simulink library "peripheral_utilities"  (R2024b)
settings: Solver=VariableStepAuto  StartTime=0.0  StopTime=10.0  RelTol=1e-3
libraries: $bdroot x19, simulink x5, spsSeriesRLCBranchLib x3, spsVoltageMeasurementLib x2, spsMosfetLib x2, spsCurrentMeasurementLib x1, spsSecondOrderFilterLib x1, spsGroundLib x1
(part 1 of 2)
settings Model: Creator=Javnson  LastModifiedBy=javnson
settings OptimizationCC: ReuseModelBlockBuffer=off
settings RTWCC: GPUComputeCapability=3.5

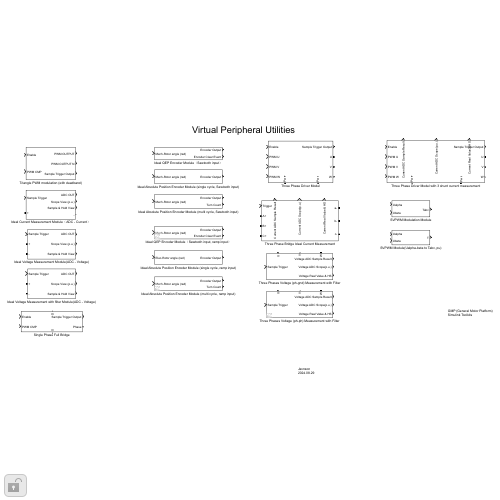
[thumbnail: Simulink's stored preview of the top-level diagram]
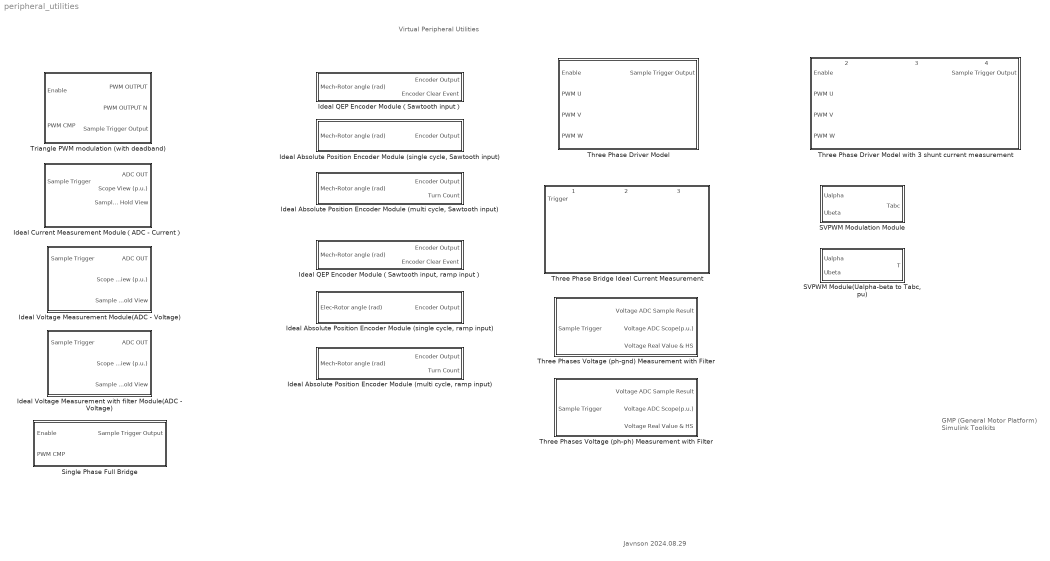
== system peripheral_utilities ==
  note: Virtual Peripheral Utilities
  note: GMP (General Motor Platform)
      | Simulink Toolkits
  note: Javnson
      | 2024.08.29
  "Ideal Absolute Position Encoder Module (multi cycle, Sawtooth input)" : Subsystem  mask{ENCODER_BIT=17}
      mask DialogControl DescGroupVar Prompt: Ideal Absolute Position Encoder Module (multi cycle, Sawtooth input)
      mask DialogControl DescTextVar Prompt: Avsolute Encoder transfer a motor mechanical angle (thetam, rad) to Absolute Encoder result. Generally, an absolute encoder has 17-bits or 23-bits resolution results.
      mask DialogControl Control3 Prompt: GMP CTL Simulink Utilities: virtual peripherals
      mask DialogControl ParameterGroupVar Prompt: 参数
      mask DialogControl Control2 Prompt: Absolute Encoder Resolution (bits):
  "Ideal Absolute Position Encoder Module (multi cycle, ramp input)" : Subsystem  AncestorBlock=peripheral_utilities/Ideal Absolute Position Encoder Module (multi cycle, Sawtooth input)  mask{ENCODER_BIT=17}
      mask DialogControl DescGroupVar Prompt: Ideal Absolute Position Encoder Module (multi cycle, Sawtooth input)
      mask DialogControl Control3 Prompt: GMP CTL Simulink Utilities: virtual peripherals
      mask DialogControl DescTextVar Prompt: Avsolute Encoder transfer a motor mechanical angle (thetam, rad) to Absolute Encoder result. Generally, an absolute encoder has 17-bits or 23-bits resolution results.
      mask DialogControl ParameterGroupVar Prompt: 参数
      mask DialogControl Control2 Prompt: Absolute Encoder Resolution (bits):
  "Ideal Absolute Position Encoder Module (single cycle, Sawtooth input)" : Subsystem  mask{ENCODER_BIT=17}
      mask DialogControl DescGroupVar Prompt: Ideal Absolute Position Encoder Module (single cycle, Sawtooth input)
      mask DialogControl DescTextVar Prompt: Avsolute Encoder transfer a motor angle (thetam, rad) to Absolute Encoder result. Generally, an absolute encoder has 17-bits or 23-bits resolution results.
      mask DialogControl Control3 Prompt: GMP CTL Simulink Utilities: virtual peripherals
      mask DialogControl ParameterGroupVar Prompt: parameters
      mask DialogControl Control2 Prompt: Absolute Encoder Resolution (bits):
  "Ideal Absolute Position Encoder Module (single cycle, ramp input)" : Subsystem  mask{ENCODER_BIT=17}
      mask DialogControl DescGroupVar Prompt: Ideal Absolute Position Encoder Module (single cycle)
      mask DialogControl DescTextVar Prompt: Avsolute Encoder transfer a motor mechanical angle (thetam, rad) to Absolute Encoder result. Generally, an absolute encoder has 17-bits or 23-bits resolution results.
      mask DialogControl Control3 Prompt: GMP CTL Simulink Utilities: virtual peripherals
      mask DialogControl ParameterGroupVar Prompt: 参数
      mask DialogControl Control2 Prompt: Absolute Encoder Resolution (bits):
  Ideal Current Measurement Module（ADC - Current） : Subsystem  mask{ADC_GAIN=1, ADC_BIT=16, ADC_REFERENCE=20.0, ADC_BIAS=10, ADC_INIT=0}
      mask DialogControl DescGroupVar Prompt: Current Sample ADC Model 1
      mask DialogControl DescTextVar Prompt: This is a ideal Current Measurement Module. This module enable a bias and a gain, and finally output a ADC result.
      mask DialogControl Control8 Prompt: ADC(p.u.) = (real_current * ADC_GAIN + ADC_BIAS)/ADC_REFERENCE
      mask DialogControl Control9 Prompt: GMP CTL Simulink Utilities: virtual peripherals
      mask DialogControl ParameterGroupVar Prompt: 参数
      mask DialogControl Control7 Prompt: ADC Current Gain (Scale Factor):
      mask DialogControl Control2 Prompt: ADC resolution:
      mask DialogControl Control4 Prompt: ADC reference Current(A), ADC full scale current (when gain = 1)
      mask DialogControl Control5 Prompt: ADC Bias Current(A)
      mask DialogControl Control6 Prompt: ADC initial Current Output(A)
  "Ideal QEP Encoder Module（Sawtooth input, ramp input）" : Subsystem  AncestorBlock=peripheral_utilities/Ideal QEP Encoder Module（Sawtooth input）  mask{QEP_LINE=2000}
      mask DialogControl DescGroupVar Prompt: Ideal QEP Encoder Module
      mask DialogControl DescTextVar Prompt: QEP encoder transfer a motor mechanical angle (thetam, rad) to QEP encoder results. The maximum output is 4 * QEP_LINE and generate a reseet event each round.
      mask DialogControl Control4 Prompt: GMP CTL Simulink Utilities: virtual peripherals
      mask DialogControl ParameterGroupVar Prompt: 参数
      mask DialogControl Control3 Prompt: QEP encoder lines count:
  Ideal QEP Encoder Module（Sawtooth input） : Subsystem  mask{QEP_LINE=2000}
      mask DialogControl DescGroupVar Prompt: Ideal QEP Encoder Module
      mask DialogControl DescTextVar Prompt: QEP encoder transfer a motor mechanical angle (thetam, rad) to QEP encoder results. The maximum output is 4 * QEP_LINE and generate a reseet event each round.
      mask DialogControl Control4 Prompt: GMP CTL Simulink Utilities: virtual peripherals
      mask DialogControl ParameterGroupVar Prompt: 参数
      mask DialogControl Control3 Prompt: QEP encoder lines count:
  Ideal Voltage Measurement Module(ADC - Voltage) : Subsystem  mask{ADC_GAIN=1/10, ADC_BIT=16, ADC_REFERENCE=3, ADC_BIAS=0, ADC_INIT=0}
      mask DialogControl DescGroupVar Prompt: Voltage Sample ADC Model
      mask DialogControl DescTextVar Prompt: This is a ideal Voltage Measurement Module.
      mask DialogControl Control2 Prompt: ADC(p.u.) = (real_voltage * ADC_GAIN + ADC_BIAS)/ADC_REFERENCE
      mask DialogControl Control9 Prompt: GMP CTL Simulink Utilities: virtual peripherals
      mask DialogControl ParameterGroupVar Prompt: Parameters:
      mask DialogControl Control4 Prompt: ADC Voltage Gain (Scale Factor):
      mask DialogControl Control5 Prompt: ADC resolution:
      mask DialogControl Control6 Prompt: ADC reference Voltage(V)
      mask DialogControl Control8 Prompt: ADC Bias Voltage(V)
      mask DialogControl Control7 Prompt: ADC Initial Voltage Output (V):
  Ideal Voltage Measurement with filter Module(ADC - Voltage) : Subsystem  mask{ADC_GAIN=1, ADC_BIT=16, ADC_REFERENCE=3, ADC_BIAS=0, ADC_INIT=0, cut_frequency=500}
      mask DialogControl DescGroupVar Prompt: Voltage Sample ADC Model
      mask DialogControl DescTextVar Prompt: This is a ideal Voltage Measurement Module.
      mask DialogControl Control2 Prompt: ADC(p.u.) = (real_voltage * ADC_GAIN + ADC_BIAS)/ADC_REFERENCE
      mask DialogControl Control11 Prompt: GMP CTL Simulink Utilities: virtual peripherals
      mask DialogControl ParameterGroupVar Prompt: Parameters:
      mask DialogControl Control4 Prompt: ADC Voltage Gain (Scale Factor):
      mask DialogControl Control5 Prompt: ADC resolution:
      mask DialogControl Control6 Prompt: ADC reference Voltage(V)
      mask DialogControl Control8 Prompt: ADC Bias Voltage(V)
      mask DialogControl Control7 Prompt: ADC Initial Voltage Output (V):
      mask DialogControl Control9 Prompt: Voltage Filter cut frequency (Hz):
      mask DialogControl Control10 Prompt: Generally, this value less than switch frequency / 10, greater than motor normal frequency * 3
  SVPWM Modulation Module : Subsystem  mask{half_cmp=10000}
      mask DialogControl DescGroupVar Prompt: SVPWM Modulation
      mask DialogControl DescTextVar Prompt: This Module Provide a dual level svpwm modulation tools.
      mask DialogControl Control4 Prompt: GMP CTL Simulink Utilities: virtual peripherals
      mask DialogControl Control3 Prompt: EPWM module Half Compare
  "SVPWM Module(Ualpha-beta to Tabc, pu)" : Subsystem  mask{half_cycle=10000}
      mask prompts: half_cycle "Half cycle"
      mask DialogControl DescGroupVar Prompt: SVPWM to Tabc
      mask DialogControl DescTextVar Prompt: GMP CTL Simulink Utilities: virtual peripherals
      mask DialogControl Control2 Prompt: SVPWM modulation module. Output is the compare register value.
      mask DialogControl ParameterGroupVar Prompt: Parameters:
      mask DialogControl Control3 Prompt: SVPWM Modulation Half cycle:
  Single Phase Full Bridge : Subsystem  mask{fswitch=10e3, CMP_MAX=10000, Deadband_Upper=100, Deadband_Lower=100, Deadband_us=1, phase_shift=0, R_mosfet_on=0.1, Lon=0, Rd=0.01, Vf=0.3, Rs=1e5, Cs=inf}
      mask init:
      | calculate_deadband(gcb, 'Deadband_Upper', 'Deadband_Lower',	'CMP_MAX', 'fswitch', 'Deadband_us');
      settings: PortSchema="{\"entries\":[{\"content\":{\"sides\":[{\"content\":{\"connectorIds\":[\"In1\",\"In2\"]},\"type\":\"ConnectorPlacement.EquallySpacedRectSide\",\"uuid\":\"20beeabc-b0ca-4337-b227-c7f02abd15d8\"},{\"content\":{\"connectorIds\":[\"Out1\",\"RConn1\"],\"side\":\"RIGHT\"},\"type\":\"ConnectorPlacement.EquallySpacedRectSide\",\"uuid\":\"a7923383-ac55-4621-ad1d-4d067c1fb84d\"},{\"content\":{\"connectorIds\":[\"LConn1\"],\"side\":\"TOP\"},\"type\":\"ConnectorPlacement.EquallySpacedRectSide\",\"uuid\":\"661bf0ae-1c96-4de8-96aa-28c06a0a56db\"},{\"content\":{\"connectorIds\":[\"RConn2\"],\"side\":\"BOTTOM\"},\"type\":\"ConnectorPlacement.EquallySpacedRectSide\",\"uuid\":\"fc2f6321-5787-4e1a-b5a2-65ed34db36b5\"}]},\"type\":\"ConnectorPlacement.EquallySpacedConnector\",\"uuid\":\"e2219b16-0a50-43ef-8183-c55a35d5a2a0\"}],\"packageUris\":[\"http://schema.mathworks.com/mf0/Connector/R2020b\"],\"version\":\"1.0\"}"
      mask Callback fswitch: calculate_deadband(gcb, 'Deadband_Upper', 'Deadband_Lower',	'CMP_MAX', 'fswitch', 'Deadband_us');
      mask Callback CMP_MAX: calculate_deadband(gcb, 'Deadband_Upper', 'Deadband_Lower',	'CMP_MAX', 'fswitch', 'Deadband_us');
      mask Callback Deadband_Upper: calculate_deadband(gcb, 'Deadband_Upper', 'Deadband_Lower',	'CMP_MAX', 'fswitch', 'Deadband_us');
      mask Callback Deadband_Lower: calculate_deadband(gcb, 'Deadband_Upper', 'Deadband_Lower',	'CMP_MAX', 'fswitch', 'Deadband_us');
      mask DialogControl DescGroupVar Prompt: Half Bridge With PWM Module
      mask DialogControl Control14 Prompt: GMP CTL Simulink Utilities: virtual peripherals
      mask DialogControl DescTextVar Prompt: This module provide a PWM (with deadband), and a MOSFET half bridge.
      mask DialogControl Container5 Prompt: PWM Modulator
      mask DialogControl ParameterGroupVar Prompt: PWM module parameters
      mask DialogControl Control2 Prompt: PWM Frequency (Hz):
      mask DialogControl Control3 Prompt: Full Scale PWM Compare value:
      mask DialogControl Control4 Prompt: (whole period is 2 * CMP_MAX ticks)
      mask DialogControl Control5 Prompt: Deadband Range Set (CMP Value):
      mask DialogControl Control6 Prompt: Single side deadband time: DEADBAND_CMP/2/CMP_MAX/fswitch
      mask DialogControl Control15 Prompt: Calculated Deadband, us
      mask DialogControl Control13 Prompt: Initial Phase Shift, unit rad
      mask DialogControl Container6 Prompt: MOSFET
      mask DialogControl Container3 Prompt: MOSFET parameters
      mask DialogControl Control7 Prompt: Rds(on), unit Ohm
      mask DialogControl Control8 Prompt: Internal diode inducctance, unit H
      mask DialogControl Control9 Prompt: Internal diode resistance Rd, unit Ohm
      mask DialogControl Control10 Prompt: Internal diode forward voltage Vf, unit V
      mask DialogControl Control11 Prompt: Snubber resistance Rs, unit ohm
      mask DialogControl Control12 Prompt: Snubber Capacitance Cs, unit F
  Three Phase Bridge Ideal Current Measurement : Subsystem  mask{ADC_GAIN=1, ADC_BIT=16, ADC_REFERENCE=50, ADC_BIAS=25, ADC_INIT=0}
      settings: PortSchema="{\"entries\":[{\"content\":{\"sides\":[{\"content\":{\"connectorIds\":[\"In1\",\"LConn1\",\"LConn2\",\"LConn3\"]},\"type\":\"ConnectorPlacement.EquallySpacedRectSide\",\"uuid\":\"b346a103-34dd-44fb-8c54-df97898fe3d3\"},{\"content\":{\"connectorIds\":[\"RConn1\",\"RConn2\",\"RConn3\"],\"side\":\"RIGHT\"},\"type\":\"ConnectorPlacement.EquallySpacedRectSide\",\"uuid\":\"8f839403-d503-4f8a-9801-ccf54d332627\"},{\"content\":{\"connectorIds\":[\"Out1\",\"Out2\",\"Out3\"],\"side\":\"TOP\"},\"type\":\"ConnectorPlacement.EquallySpacedRectSide\",\"uuid\":\"85557c89-7bb0-4df8-9b93-9dbb31201649\"}]},\"type\":\"ConnectorPlacement.EquallySpacedConnector\",\"uuid\":\"64a00c7b-bd9b-45ba-9c15-20a815983bbc\"}],\"packageUris\":[\"http://schema.mathworks.com/mf0/Connector/R2020b\"],\"version\":\"1.0\"}"
      mask DialogControl DescGroupVar Prompt: Current Sample ADC Module 3 phases
      mask DialogControl Control7 Prompt: GMP CTL Simulink Utilities: virtual peripherals
      mask DialogControl DescTextVar Prompt: This is a ideal Current Measurement Module. This module enable a bias and a gain, and finally output a ADC result.
      mask DialogControl ParameterGroupVar Prompt: parameter
      mask DialogControl Control2 Prompt: ADC Current Gain (Scale Factor):
      mask DialogControl Control3 Prompt: ADC resolution:
      mask DialogControl Control4 Prompt: ADC reference Current (A), ADC full scale current (when gain = 1)
      mask DialogControl Control5 Prompt: ADC Bias Current(A)
      mask DialogControl Control6 Prompt: ADC initial Current Output(A)
  Three Phase Driver Model : Subsystem  mask{fswitch=10e3, CMP_MAX=10000, Deadband_Upper=100, Deadband_Lower=100, phase_shift=0, R_mosfet_on=0.1, Lon=0, Rd=0.01, Vf=0.3, Rs=1e5, Cs=inf}
      settings: PortSchema="{\"entries\":[{\"content\":{\"sides\":[{\"content\":{\"connectorIds\":[\"In1\",\"In2\",\"In3\",\"In4\"]},\"type\":\"ConnectorPlacement.EquallySpacedRectSide\",\"uuid\":\"3ffcf095-7a60-4897-81b4-d3692ae6e2ab\"},{\"content\":{\"connectorIds\":[\"Out1\",\"RConn1\",\"RConn2\",\"RConn3\"],\"side\":\"RIGHT\"},\"type\":\"ConnectorPlacement.EquallySpacedRectSide\",\"uuid\":\"6e5cf4cf-b1b9-48ac-a692-0a8874277a23\"},{\"content\":{\"connectorIds\":[],\"side\":\"TOP\"},\"type\":\"ConnectorPlacement.EquallySpacedRectSide\",\"uuid\":\"9aa765f5-1b2f-406c-a04a-fab38ac2c4f7\"},{\"content\":{\"connectorIds\":[\"RConn4\",\"RConn5\"],\"side\":\"BOTTOM\"},\"type\":\"ConnectorPlacement.EquallySpacedRectSide\",\"uuid\":\"ff3856e6-d154-4ba2-8db0-f3c94a45cad8\"}]},\"type\":\"ConnectorPlacement.EquallySpacedConnector\",\"uuid\":\"490a993e-7d06-4faf-ab4a-bafd9b6172f2\"}],\"packageUris\":[\"http://schema.mathworks.com/mf0/Connector/R2020b\"],\"version\":\"1.0\"}"
      mask DialogControl DescGroupVar Prompt: Three Phases Bridge Peripheral
      mask DialogControl Control15 Prompt: GMP CTL Simulink Utilities: virtual peripherals
      mask DialogControl DescTextVar Prompt: This module provide a ideal 3-phases bridge peripheral.
      mask DialogControl Container5 Prompt: PWM Modulator
      mask DialogControl ParameterGroupVar Prompt: PWM module parameters
      mask DialogControl Control2 Prompt: PWM Frequency (Hz):
      mask DialogControl Control3 Prompt: Full Scale PWM Compare value:
      mask DialogControl Control5 Prompt: Deadband Range Set (CMP Value):
      mask DialogControl Control6 Prompt: Deadband time: DEADBAND_CMP/2/CMP_MAX/fswitch
      mask DialogControl Control4 Prompt: (whole period is 2 * CMP_MAX ticks)
      mask DialogControl Control14 Prompt: Initial Phase Shift, unit rad
      mask DialogControl Container6 Prompt: MOSFET
      mask DialogControl Container3 Prompt: MOSFET parameters
      mask DialogControl Control7 Prompt: Rds(on), unit Ohm
      mask DialogControl Control8 Prompt: Internal diode inducctance, unit H
      mask DialogControl Control9 Prompt: Internal diode resistance Rd, unit Ohm
      mask DialogControl Control10 Prompt: Internal diode forward voltage Vf, unit V
      mask DialogControl Control11 Prompt: Snubber resistance Rs, unit ohm
      mask DialogControl Control13 Prompt: Snubber Capacitance Cs, unit F
  Three Phase Driver Model with 3 shunt current measurement : Subsystem  mask{fswitch=10e3, CMP_MAX=10000, Deadband_Upper=100, Deadband_Lower=100, Deadband_us=1, phase_shift=0, R_mosfet_on=0.1, Lon=0, Rd=0.01, Vf=0.3, Rs=1e5, Cs=inf, Rsap=0.1, ADC_GAIN=0.1, ADC_BIT=16, ADC_REFERENCE=3.0, ADC_BIAS=1.5, ADC_INIT=0}
      mask init:
      | calculate_deadband(gcb, 'Deadband_Upper', 'Deadband_Lower',	'CMP_MAX', 'fswitch', 'Deadband_us');
      settings: PortSchema="{\"entries\":[{\"content\":{\"sides\":[{\"content\":{\"connectorIds\":[\"In1\",\"In2\",\"In3\",\"In4\"]},\"type\":\"ConnectorPlacement.EquallySpacedRectSide\",\"uuid\":\"3f4c86ad-0582-4f47-8583-a8af9a7f9adc\"},{\"content\":{\"connectorIds\":[\"Out1\",\"RConn1\",\"RConn2\",\"RConn3\"],\"side\":\"RIGHT\"},\"type\":\"ConnectorPlacement.EquallySpacedRectSide\",\"uuid\":\"ae91f325-3014-4188-9063-296f4d5623fa\"},{\"content\":{\"connectorIds\":[\"Out2\",\"Out3\",\"Out4\"],\"side\":\"TOP\"},\"type\":\"ConnectorPlacement.EquallySpacedRectSide\",\"uuid\":\"5f2edb36-6849-4a72-b7bd-4d267f120ce4\"},{\"content\":{\"connectorIds\":[\"RConn4\",\"RConn5\"],\"side\":\"BOTTOM\"},\"type\":\"ConnectorPlacement.EquallySpacedRectSide\",\"uuid\":\"79a111ed-6591-4ced-9242-67ea1247c580\"}]},\"type\":\"ConnectorPlacement.EquallySpacedConnector\",\"uuid\":\"8c66eb8e-d25c-472f-a4a5-d1759225ba1c\"}],\"packageUris\":[\"http://schema.mathworks.com/mf0/Connector/R2020b\"],\"version\":\"1.0\"}"
      mask Callback fswitch: calculate_deadband(gcb, 'Deadband_Upper', 'Deadband_Lower',	'CMP_MAX', 'fswitch', 'Deadband_us');
      mask Callback CMP_MAX: calculate_deadband(gcb, 'Deadband_Upper', 'Deadband_Lower',	'CMP_MAX', 'fswitch', 'Deadband_us');
      mask Callback Deadband_Upper: calculate_deadband(gcb, 'Deadband_Upper', 'Deadband_Lower',	'CMP_MAX', 'fswitch', 'Deadband_us');
      mask Callback Deadband_Lower: calculate_deadband(gcb, 'Deadband_Upper', 'Deadband_Lower',	'CMP_MAX', 'fswitch', 'Deadband_us');
      mask DialogControl DescGroupVar Prompt: Three Phases Bridge Peripheral(3-shunt sample)
      mask DialogControl Control21 Prompt: GMP CTL Simulink Utilities: virtual peripherals
      mask DialogControl DescTextVar Prompt: This module provide a ideal 3-phases bridge peripheral.
      mask DialogControl Container4 Prompt: PWM config
      mask DialogControl ParameterGroupVar Prompt: PWM parameters
      mask DialogControl Control2 Prompt: PWM Frequency (Hz):
      mask DialogControl Control4 Prompt: Full Scale PWM Compare value:
      mask DialogControl Control5 Prompt: Deadband Range Set (CMP Value):
      mask DialogControl Control6 Prompt: Deadband time: DEADBAND_CMP/2/CMP_MAX/fswitch
      mask DialogControl Control22 Prompt: Calculated Deadband, us
      mask DialogControl Control20 Prompt: Initial Phase shift:
      mask DialogControl Container5 Prompt: MOSFET config
      mask DialogControl Container7 Prompt: MOSFET parameters
      mask DialogControl Control7 Prompt: Rds(on), unit Ohm
      mask DialogControl Control8 Prompt: Internal diode inducctance, unit H
      mask DialogControl Control9 Prompt: Internal diode resistance Rd, unit Ohm
      mask DialogControl Control10 Prompt: Internal diode forward voltage Vf, unit V
      mask DialogControl Control11 Prompt: Snubber resistance Rs, unit ohm
      mask DialogControl Control12 Prompt: Snubber Capacitance Cs, unit F
      mask DialogControl Container6 Prompt: 3-shunt current sample
      mask DialogControl Control13 Prompt: ADC(p.u.) = (real_voltage * ADC_GAIN + ADC_BIAS)/ADC_REFERENCE
      mask DialogControl Control15 Prompt: Shunt Smaple Res, unit Ohm
      mask DialogControl Control14 Prompt: ADC Voltage Gain (Scale Factor):
      mask DialogControl Control16 Prompt: ADC resolution:
      mask DialogControl Control17 Prompt: ADC reference Voltage(V)
      mask DialogControl Control18 Prompt: ADC Bias Voltage(V)
      mask DialogControl Control19 Prompt: ADC Initial Voltage Output (V):
  Three Phases Voltage (ph-gnd) Measurement with Filter : Subsystem  mask{ADC_GAIN=1, ADC_BIT=16, ADC_REFERENCE=48, ADC_BIAS=24, ADC_INIT=0, cut_frequency=500}
      settings: PortSchema="{\"entries\":[{\"content\":{\"sides\":[{\"content\":{\"connectorIds\":[\"In1\"]},\"type\":\"ConnectorPlacement.EquallySpacedRectSide\",\"uuid\":\"ae4f4612-c092-4fa0-8a43-5c9e823110e3\"},{\"content\":{\"connectorIds\":[\"Out1\",\"Out2\",\"Out3\"],\"side\":\"RIGHT\"},\"type\":\"ConnectorPlacement.EquallySpacedRectSide\",\"uuid\":\"6db15ef0-d33a-4775-b4e6-14a566796673\"},{\"content\":{\"connectorIds\":[\"LConn1\",\"LConn2\",\"LConn3\"],\"side\":\"TOP\"},\"type\":\"ConnectorPlacement.EquallySpacedRectSide\",\"uuid\":\"cfddd664-59f3-497b-b33e-fe832fe7a7bd\"}]},\"type\":\"ConnectorPlacement.EquallySpacedConnector\",\"uuid\":\"5bacf0ad-0c4a-4f47-a242-d8a476ab7f52\"}],\"packageUris\":[\"http://schema.mathworks.com/mf0/Connector/R2020b\"],\"version\":\"1.0\"}"
      mask DialogControl DescGroupVar Prompt: 3 phases Voltage Sample ADC Model
      mask DialogControl Control10 Prompt: GMP CTL Simulink Utilities: virtual peripherals
      mask DialogControl DescTextVar Prompt: This is a ideal Voltage Measurement Module.
      mask DialogControl Control2 Prompt: ADC(p.u.) = (real_voltage * ADC_GAIN + ADC_BIAS)/ADC_REFERENCE
      mask DialogControl ParameterGroupVar Prompt: parameters:
      mask DialogControl Control3 Prompt: ADC Voltage Gain (Scale Factor):
      mask DialogControl Control4 Prompt: ADC resolution:
      mask DialogControl Control5 Prompt: ADC reference Voltage (V), when ADC_GAIN=1, ADC_REF = ADC full scale
      mask DialogControl Control6 Prompt: ADC Bias Voltage(V)
      mask DialogControl Control7 Prompt: ADC Initial Voltage Output (V):
      mask DialogControl Control8 Prompt: Voltage Filter cut frequency (Hz):
      mask DialogControl Control9 Prompt: Generally, this value less than switch frequency / 10, greater than motor normal frequency * 3
  Three Phases Voltage (ph-ph) Measurement with Filter : Subsystem  AncestorBlock=peripheral_utilities/Three Phases Voltage (ph-gnd) Measurement with Filter  mask{ADC_GAIN=1, ADC_BIT=16, ADC_REFERENCE=48, ADC_BIAS=24, ADC_INIT=0, cut_frequency=500}
      settings: PortSchema="{\"entries\":[{\"content\":{\"sides\":[{\"content\":{\"connectorIds\":[\"In1\"]},\"type\":\"ConnectorPlacement.EquallySpacedRectSide\",\"uuid\":\"ae4f4612-c092-4fa0-8a43-5c9e823110e3\"},{\"content\":{\"connectorIds\":[\"Out1\",\"Out2\",\"Out3\"],\"side\":\"RIGHT\"},\"type\":\"ConnectorPlacement.EquallySpacedRectSide\",\"uuid\":\"6db15ef0-d33a-4775-b4e6-14a566796673\"},{\"content\":{\"connectorIds\":[\"LConn1\",\"LConn2\",\"LConn3\"],\"side\":\"TOP\"},\"type\":\"ConnectorPlacement.EquallySpacedRectSide\",\"uuid\":\"cfddd664-59f3-497b-b33e-fe832fe7a7bd\"}]},\"type\":\"ConnectorPlacement.EquallySpacedConnector\",\"uuid\":\"5bacf0ad-0c4a-4f47-a242-d8a476ab7f52\"}],\"packageUris\":[\"http://schema.mathworks.com/mf0/Connector/R2020b\"],\"version\":\"1.0\"}"
      mask DialogControl DescGroupVar Prompt: 3 phases Voltage Sample ADC Model
      mask DialogControl DescTextVar Prompt: This is a ideal Voltage Measurement Module.
      mask DialogControl Control2 Prompt: ADC(p.u.) = (real_voltage * ADC_GAIN + ADC_BIAS)/ADC_REFERENCE
      mask DialogControl Control10 Prompt: GMP CTL Simulink Utilities: virtual peripherals
      mask DialogControl ParameterGroupVar Prompt: parameters:
      mask DialogControl Control3 Prompt: ADC Voltage Gain (Scale Factor):
      mask DialogControl Control4 Prompt: ADC resolution:
      mask DialogControl Control5 Prompt: ADC reference Voltage (V), when ADC_GAIN=1, ADC_REF = ADC full scale
      mask DialogControl Control6 Prompt: ADC Bias Voltage(V)
      mask DialogControl Control7 Prompt: ADC Initial Voltage Output (V):
      mask DialogControl Control8 Prompt: Voltage Filter cut frequency (Hz):
      mask DialogControl Control9 Prompt: Generally, this value less than switch frequency / 10, greater than motor normal frequency * 3
  Triangle PWM modulation (with deadband) : Subsystem  mask{fswitch=10e3, CMP_MAX=2000, Deadband_Upper=200, Deadband_Lower=100, Deadband_us=[], phase_shift=0}
      mask prompts: Deadband_us "Deadband Time: (μs)"
      mask init:
      | calculate_deadband(gcb, 'Deadband_Upper', 'Deadband_Lower',	'CMP_MAX', 'fswitch', 'Deadband_us');
      mask Callback fswitch: calculate_deadband(gcb, 'Deadband_Upper', 'Deadband_Lower',	'CMP_MAX', 'fswitch', 'Deadband_us');
      mask Callback CMP_MAX: calculate_deadband(gcb, 'Deadband_Upper', 'Deadband_Lower',	'CMP_MAX', 'fswitch', 'Deadband_us');
      mask Callback Deadband_Upper:
      | calculate_deadband(gcb, 'Deadband_Upper', 'Deadband_Lower',	'CMP_MAX', 'fswitch', 'Deadband_us');
      | 
      | % Get handle of Mask
      | %mask_obj = Simulink.Mask.get(gcb);
      | %Parameters = Simulink.Mask.get(gcb).Parameters;
      | 
      | % Get source data
      | %dead_band_up = str2double(Parameters(strcmp(get_param(gcb,'MaskNames'),'Deadband_Upper')==1).Value);
      | %dead_band_dn = str2double(Parameters(strcmp(get_param(gcb,'MaskNames'),'Deadband_Lower')==1).Value);
      | %cmp_max = str2double(Parameters(strcmp(get_param(gcb,'MaskNames'),'CMP_MAX')==1).Value);
      | %switch_freq = str2double(Parameters(strcmp(get_param(gcb,'MaskNames'),'fswitch')==1).Value);
      | 
      | % calculate deadband
      | %dead_band_us = 1/switch_freq * (dead_band_up + dead_band_dn) / cmp_max*1e6;
      | 
      | % Set result
      | %Parameters(strcmp(get_param(gcb,'MaskNames'),'Deadband_upper_us')==1).Value=num2str(dead_band_us);
      mask Callback Deadband_Lower: calculate_deadband(gcb, 'Deadband_Upper', 'Deadband_Lower',	'CMP_MAX', 'fswitch', 'Deadband_upper_us');
      mask DialogControl DescGroupVar Prompt: PWM Modulator
      mask DialogControl Control8 Prompt: GMP CTL Simulink Utilities: virtual peripherals
      mask DialogControl DescTextVar Prompt: PWM Modulator. Input PWM compare register value, output ADC trigger signal, PWM output and negtive PWM output.
      mask DialogControl ParameterGroupVar Prompt: 参数
      mask DialogControl Control2 Prompt: PWM Frequency (Hz) :
      mask DialogControl Control4 Prompt: Full Scale PWM Compare value:
      mask DialogControl Control5 Prompt: (whole period is 2 * CMP_MAX ticks)
      mask DialogControl Control3 Prompt: Deadband Range Set (CMP Value):
      mask DialogControl Control6 Prompt: Single side deadband time: DEADBAND_CMP/2/CMP_MAX/fswitch
      mask DialogControl Control7 Prompt: Initial Phase (rad)

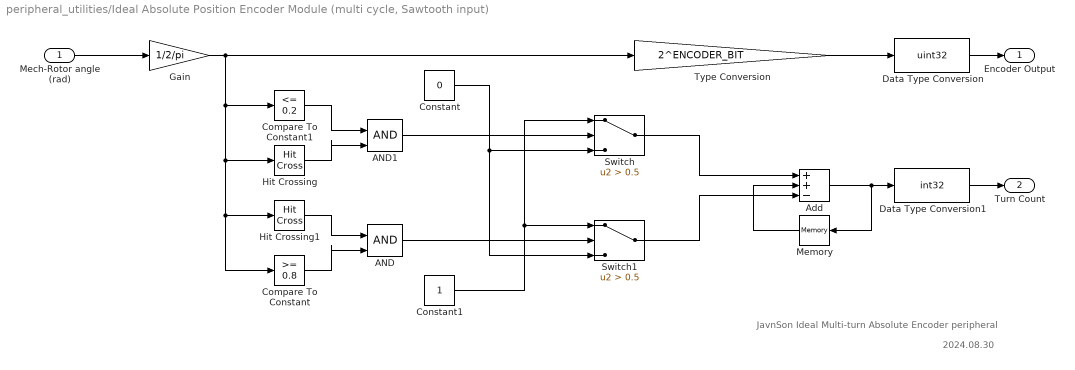
== system peripheral_utilities/Ideal Absolute Position Encoder Module (multi cycle, Sawtooth input) ==
  note: JavnSon Ideal Multi-turn Absolute Encoder peripheral
  note: 2024.08.30
  Mech-Rotor angle (rad) : Inport
  AND : Logic  IconShape=distinctive  AllPortsSameDT=off  OutDataTypeStr=boolean
  AND1 : Logic  IconShape=distinctive  AllPortsSameDT=off  OutDataTypeStr=boolean
  Add : Sum  Inputs=++-
  Compare To Constant : simulink/Logic and Bit Operations/Compare To Constant  relop=>=  const=0.8  OutDataTypeStr=boolean
  Compare To Constant1 : simulink/Logic and Bit Operations/Compare To Constant  relop=<=  const=0.2  OutDataTypeStr=boolean
  Constant : Constant  Value=0
  Constant1 : Constant
  Data Type Conversion : DataTypeConversion  OutDataTypeStr=uint32  SaturateOnIntegerOverflow=off  RndMeth=Floor
  Data Type Conversion1 : DataTypeConversion  OutDataTypeStr=int32  SaturateOnIntegerOverflow=off  RndMeth=Floor
  Gain : Gain  Gain=1/2/pi
  Hit Crossing : HitCross  HitCrossingOffset=0.5  HitCrossingDirection=falling
  Hit Crossing1 : HitCross  HitCrossingOffset=0.5  HitCrossingDirection=rising
  Memory : Memory
  Switch : Switch  Criteria=u2 > Threshold  Threshold=0.5  SaturateOnIntegerOverflow=off  InputSameDT=off
  Switch1 : Switch  Criteria=u2 > Threshold  Threshold=0.5  SaturateOnIntegerOverflow=off  InputSameDT=off
  Type Conversion : Gain  Gain=2^ENCODER_BIT
  Encoder Output : Outport
  Turn Count : Outport  Port=2
  wires:
  Gain/1 -> Compare To Constant1/1, Hit Crossing/1, Compare To Constant/1, Hit Crossing1/1, Type Conversion/1
  Type Conversion/1 -> Data Type Conversion/1
  Data Type Conversion/1 -> Encoder Output/1
  Mech-Rotor angle (rad)/1 -> Gain/1
  Memory/1 -> Add/2
  Add/1 -> Data Type Conversion1/1, Memory/1
  Switch/1 -> Add/1
  Hit Crossing1/1 -> AND/1
  Data Type Conversion1/1 -> Turn Count/1
  Switch1/1 -> Add/3
  Compare To Constant/1 -> AND/2
  AND/1 -> Switch1/2
  Hit Crossing/1 -> AND1/2
  Compare To Constant1/1 -> AND1/1
  AND1/1 -> Switch/2
  Constant1/1 -> Switch1/1, Switch/1
  Constant/1 -> Switch1/3, Switch/3

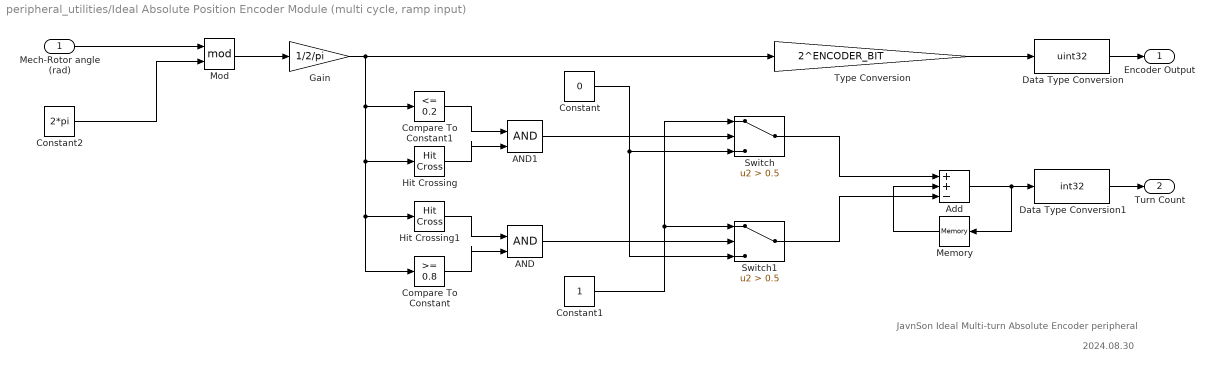
== system peripheral_utilities/Ideal Absolute Position Encoder Module (multi cycle, ramp input) ==
  note: JavnSon Ideal Multi-turn Absolute Encoder peripheral
  note: 2024.08.30
  Mech-Rotor angle (rad) : Inport
  AND : Logic  IconShape=distinctive  AllPortsSameDT=off  OutDataTypeStr=boolean
  AND1 : Logic  IconShape=distinctive  AllPortsSameDT=off  OutDataTypeStr=boolean
  Add : Sum  Inputs=++-
  Compare To Constant : simulink/Logic and Bit Operations/Compare To Constant  relop=>=  const=0.8  OutDataTypeStr=boolean
  Compare To Constant1 : simulink/Logic and Bit Operations/Compare To Constant  relop=<=  const=0.2  OutDataTypeStr=boolean
  Constant : Constant  Value=0
  Constant1 : Constant
  Constant2 : Constant  Value=2*pi
  Data Type Conversion : DataTypeConversion  OutDataTypeStr=uint32  SaturateOnIntegerOverflow=off  RndMeth=Floor
  Data Type Conversion1 : DataTypeConversion  OutDataTypeStr=int32  SaturateOnIntegerOverflow=off  RndMeth=Floor
  Gain : Gain  Gain=1/2/pi
  Hit Crossing : HitCross  HitCrossingOffset=0.5  HitCrossingDirection=falling
  Hit Crossing1 : HitCross  HitCrossingOffset=0.5  HitCrossingDirection=rising
  Memory : Memory
  Mod : Math  Operator=mod
  Switch : Switch  Criteria=u2 > Threshold  Threshold=0.5  SaturateOnIntegerOverflow=off  InputSameDT=off
  Switch1 : Switch  Criteria=u2 > Threshold  Threshold=0.5  SaturateOnIntegerOverflow=off  InputSameDT=off
  Type Conversion : Gain  Gain=2^ENCODER_BIT
  Encoder Output : Outport
  Turn Count : Outport  Port=2
  wires:
  Gain/1 -> Compare To Constant1/1, Hit Crossing/1, Compare To Constant/1, Hit Crossing1/1, Type Conversion/1
  Type Conversion/1 -> Data Type Conversion/1
  Data Type Conversion/1 -> Encoder Output/1
  Memory/1 -> Add/2
  Add/1 -> Data Type Conversion1/1, Memory/1
  Switch/1 -> Add/1
  Hit Crossing1/1 -> AND/1
  Data Type Conversion1/1 -> Turn Count/1
  Switch1/1 -> Add/3
  Compare To Constant/1 -> AND/2
  AND/1 -> Switch1/2
  Hit Crossing/1 -> AND1/2
  Compare To Constant1/1 -> AND1/1
  AND1/1 -> Switch/2
  Constant1/1 -> Switch1/1, Switch/1
  Constant/1 -> Switch1/3, Switch/3
  Mod/1 -> Gain/1
  Constant2/1 -> Mod/2
  Mech-Rotor angle (rad)/1 -> Mod/1

== system peripheral_utilities/Ideal Absolute Position Encoder Module (single cycle, Sawtooth input) ==
  note: 2024.08.30
  note: JavnSon Ideal Absolute Encoder peripheral
  Mech-Rotor angle (rad) : Inport
  Data Type Conversion : DataTypeConversion  OutDataTypeStr=uint32  SaturateOnIntegerOverflow=off  RndMeth=Floor
  Gain : Gain  Gain=1/2/pi
  Type Conversion : Gain  Gain=2^ENCODER_BIT
  Encoder Output : Outport
  wires:
  Gain/1 -> Type Conversion/1
  Type Conversion/1 -> Data Type Conversion/1
  Data Type Conversion/1 -> Encoder Output/1
  Mech-Rotor angle (rad)/1 -> Gain/1

== system peripheral_utilities/Ideal Absolute Position Encoder Module (single cycle, ramp input) ==
  Elec-Rotor angle (rad) : Inport
  Constant : Constant  Value=2*pi
  Data Type Conversion : DataTypeConversion  OutDataTypeStr=uint32  SaturateOnIntegerOverflow=off  RndMeth=Floor
  Gain : Gain  Gain=1/2/pi
  Mod : Math  Operator=mod
  Type Conversion : Gain  Gain=2^ENCODER_BIT
  Encoder Output : Outport
  wires:
  Gain/1 -> Type Conversion/1
  Type Conversion/1 -> Data Type Conversion/1
  Data Type Conversion/1 -> Encoder Output/1
  Elec-Rotor angle (rad)/1 -> Mod/1
  Mod/1 -> Gain/1
  Constant/1 -> Mod/2

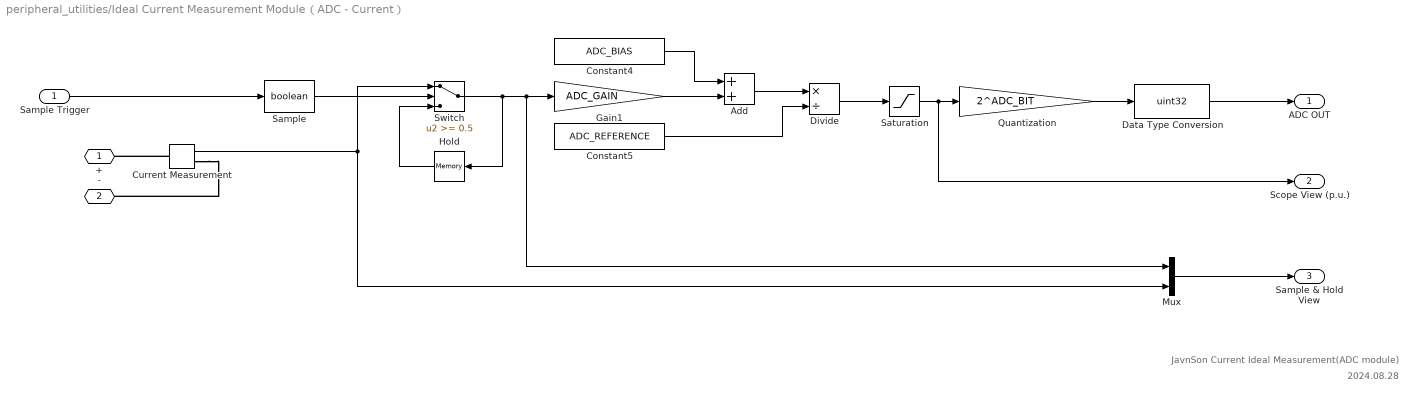
== system peripheral_utilities/Ideal Current Measurement Module（ADC - Current） ==
  note: JavnSon Current Ideal Measurement(ADC module)
  note: 2024.08.28
  Sample Trigger : Inport
  Add : Sum
  Constant4 : Constant  Value=ADC_BIAS
  Constant5 : Constant  Value=ADC_REFERENCE
  Current Measurement : spsCurrentMeasurementLib/Current Measurement  PhasorSimulation=off  OutputType=Complex  PSBequivalent=0
  Data Type Conversion : DataTypeConversion  OutDataTypeStr=uint32  ConvertRealWorld=Stored Integer (SI)  SaturateOnIntegerOverflow=off  RndMeth=Floor
  Divide : Product  Inputs=*/
  Gain1 : Gain  Gain=ADC_GAIN
  Hold : Memory  InitialCondition=ADC_INIT  LinearizeAsDelay=on
  Mux : Mux  Inputs=2
  Quantization : Gain  Gain=2^ADC_BIT
  Sample : DataTypeConversion  OutDataTypeStr=boolean  SaturateOnIntegerOverflow=off  RndMeth=Floor
  Saturation : Saturate  UpperLimit=1  LowerLimit=0
  Switch : Switch  Threshold=0.5
  + : PMIOPort  Side=Left
  - : PMIOPort  Port=2  Side=Right
  ADC OUT : Outport
  Scope View (p.u.) : Outport  Port=2
  Sample & Hold View : Outport  Port=3
  wires:
  Constant5/1 -> Divide/2
  Quantization/1 -> Data Type Conversion/1
  Sample/1 -> Switch/2
  Add/1 -> Divide/1
  Sample Trigger/1 -> Sample/1
  Data Type Conversion/1 -> ADC OUT/1
  Hold/1 -> Switch/3
  Current Measurement/1 -> Mux/2, Switch/1
  Constant4/1 -> Add/1
  Switch/1 -> Hold/1, Mux/1, Gain1/1
  Gain1/1 -> Add/2
  Saturation/1 -> Scope View (p.u.)/1, Quantization/1
  Divide/1 -> Saturation/1
  Mux/1 -> Sample & Hold View/1
  connections:
  Current Measurement/LConn1 -- +/RConn1
  Current Measurement/RConn1 -- -/RConn1

== system peripheral_utilities/Ideal QEP Encoder Module（Sawtooth input, ramp input） ==
  note: JavnSon Ideal QEP peripheral
  note: 2024.08.30
  Mech-Rotor angle (rad) : Inport
  Constant2 : Constant  Value=2*pi
  Data Type Conversion : DataTypeConversion  OutDataTypeStr=uint32  SaturateOnIntegerOverflow=off  RndMeth=Floor
  Gain : Gain  Gain=1/2/pi
  Hit Crossing : HitCross  HitCrossingDirection=rising
  Hit Crossing1 : HitCross  HitCrossingOffset=1  HitCrossingDirection=falling
  Mod : Math  Operator=mod
  OR : Logic  Operator=OR  IconShape=distinctive  AllPortsSameDT=off  OutDataTypeStr=boolean
  Type Conversion : Gain  Gain=4*QEP_LINE
  Encoder Output : Outport
  Encoder Clear Event : Outport  Port=2
  wires:
  Data Type Conversion/1 -> Encoder Output/1
  Type Conversion/1 -> Data Type Conversion/1
  Gain/1 -> Hit Crossing1/1, Hit Crossing/1, Type Conversion/1
  OR/1 -> Encoder Clear Event/1
  Hit Crossing/1 -> OR/1
  Hit Crossing1/1 -> OR/2
  Mech-Rotor angle (rad)/1 -> Mod/1
  Mod/1 -> Gain/1
  Constant2/1 -> Mod/2

== system peripheral_utilities/Ideal QEP Encoder Module（Sawtooth input） ==
  note: JavnSon Ideal QEP peripheral
  note: 2024.08.30
  Mech-Rotor angle (rad) : Inport
  Data Type Conversion : DataTypeConversion  OutDataTypeStr=uint32  SaturateOnIntegerOverflow=off  RndMeth=Floor
  Gain : Gain  Gain=1/2/pi
  Hit Crossing : HitCross  HitCrossingDirection=rising
  Hit Crossing1 : HitCross  HitCrossingOffset=1  HitCrossingDirection=falling
  OR : Logic  Operator=OR  IconShape=distinctive  AllPortsSameDT=off  OutDataTypeStr=boolean
  Type Conversion : Gain  Gain=4*QEP_LINE
  Encoder Output : Outport
  Encoder Clear Event : Outport  Port=2
  wires:
  Mech-Rotor angle (rad)/1 -> Gain/1
  Data Type Conversion/1 -> Encoder Output/1
  Type Conversion/1 -> Data Type Conversion/1
  Gain/1 -> Hit Crossing1/1, Hit Crossing/1, Type Conversion/1
  OR/1 -> Encoder Clear Event/1
  Hit Crossing/1 -> OR/1
  Hit Crossing1/1 -> OR/2

== system peripheral_utilities/Ideal Voltage Measurement Module(ADC - Voltage) ==
  note: JavnSon Voltage Ideal Measurement(ADC module)
  note: 2024.08.28
  Sample Trigger : Inport
  Add : Sum
  Constant4 : Constant  Value=ADC_BIAS
  Constant5 : Constant  Value=ADC_REFERENCE
  Data Type Conversion : DataTypeConversion  OutDataTypeStr=uint32  ConvertRealWorld=Stored Integer (SI)  SaturateOnIntegerOverflow=off  RndMeth=Floor
  Divide : Product  Inputs=*/
  Gain1 : Gain  Gain=ADC_GAIN
  Hold : Memory  InitialCondition=ADC_INIT  LinearizeAsDelay=on
  Mux1 : Mux  Inputs=2
  Quantization : Gain  Gain=2^ADC_BIT
  Sample : DataTypeConversion  OutDataTypeStr=boolean  SaturateOnIntegerOverflow=off  RndMeth=Floor
  Saturation : Saturate  UpperLimit=1  LowerLimit=0
  Switch : Switch  Threshold=0.5
  Voltage Measurement : spsVoltageMeasurementLib/Voltage Measurement  PhasorSimulation=off  OutputType=Complex  PSBequivalent=0
  + : PMIOPort  Side=Left
  - : PMIOPort  Port=2  Side=Left
  ADC OUT : Outport
  Scope View (p.u.) : Outport  Port=2
  Sample & Hold View : Outport  Port=3
  wires:
  Hold/1 -> Switch/3
  Switch/1 -> Hold/1, Mux1/1, Gain1/1
  Divide/1 -> Saturation/1
  Voltage Measurement/1 -> Mux1/2, Switch/1
  Saturation/1 -> Scope View (p.u.)/1, Quantization/1
  Constant4/1 -> Add/1
  Gain1/1 -> Add/2
  Sample Trigger/1 -> Sample/1
  Data Type Conversion/1 -> ADC OUT/1
  Mux1/1 -> Sample & Hold View/1
  Quantization/1 -> Data Type Conversion/1
  Constant5/1 -> Divide/2
  Add/1 -> Divide/1
  Sample/1 -> Switch/2
  connections:
  Voltage Measurement/LConn1 -- +/RConn1
  Voltage Measurement/LConn2 -- -/RConn1

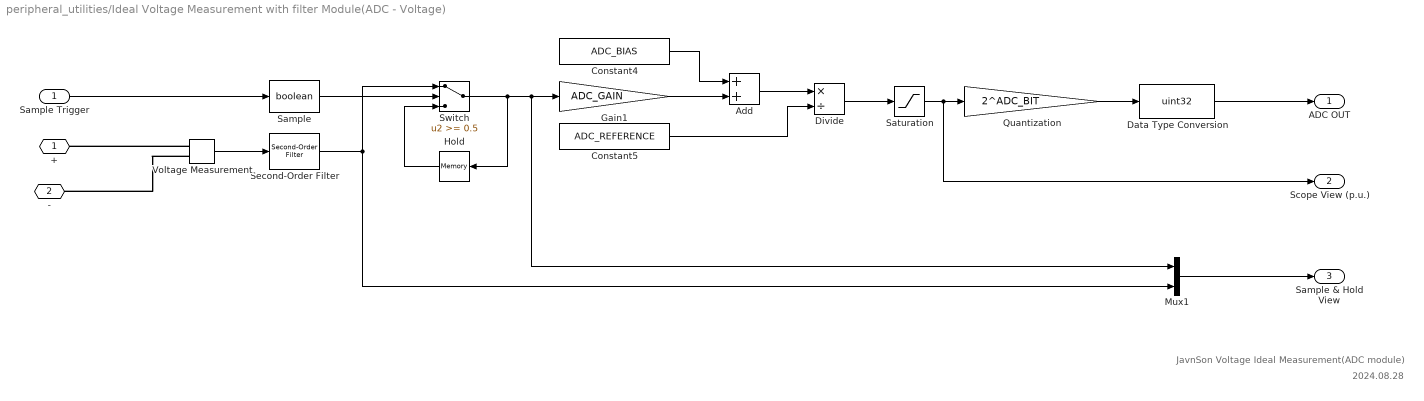
== system peripheral_utilities/Ideal Voltage Measurement with filter Module(ADC - Voltage) ==
  note: 2024.08.28
  note: JavnSon Voltage Ideal Measurement(ADC module)
  Sample Trigger : Inport
  Add : Sum
  Constant4 : Constant  Value=ADC_BIAS
  Constant5 : Constant  Value=ADC_REFERENCE
  Data Type Conversion : DataTypeConversion  OutDataTypeStr=uint32  ConvertRealWorld=Stored Integer (SI)  SaturateOnIntegerOverflow=off  RndMeth=Floor
  Divide : Product  Inputs=*/
  Gain1 : Gain  Gain=ADC_GAIN
  Hold : Memory  InitialCondition=ADC_INIT  LinearizeAsDelay=on
  Mux1 : Mux  Inputs=2
  Quantization : Gain  Gain=2^ADC_BIT
  Sample : DataTypeConversion  OutDataTypeStr=boolean  SaturateOnIntegerOverflow=off  RndMeth=Floor
  Saturation : Saturate  UpperLimit=1  LowerLimit=0
  Second-Order Filter : spsSecondOrderFilterLib/Second-Order Filter  FilterType=Lowpass  Fo=cut_frequency  Zeta=0.707  Ts=0  Initialize=off  Vac_Init="[0,  0,  60]"  Vdc_Init=0  PlotResponse=off  FreqRange=[0, 500, 1]
      settings: LibrarySourceBlock=|
      | sps_lib/Control/Filters/Second-Order
      | Filter
  Switch : Switch  Threshold=0.5
  Voltage Measurement : spsVoltageMeasurementLib/Voltage Measurement  PhasorSimulation=off  OutputType=Complex  PSBequivalent=0
  + : PMIOPort  Side=Left
  - : PMIOPort  Port=2  Side=Left
  ADC OUT : Outport
  Scope View (p.u.) : Outport  Port=2
  Sample & Hold View : Outport  Port=3
  wires:
  Sample/1 -> Switch/2
  Add/1 -> Divide/1
  Constant5/1 -> Divide/2
  Quantization/1 -> Data Type Conversion/1
  Mux1/1 -> Sample & Hold View/1
  Data Type Conversion/1 -> ADC OUT/1
  Sample Trigger/1 -> Sample/1
  Gain1/1 -> Add/2
  Constant4/1 -> Add/1
  Saturation/1 -> Quantization/1, Scope View (p.u.)/1
  Voltage Measurement/1 -> Second-Order Filter/1
  Divide/1 -> Saturation/1
  Switch/1 -> Gain1/1, Mux1/1, Hold/1
  Hold/1 -> Switch/3
  Second-Order Filter/1 -> Switch/1, Mux1/2
  connections:
  Voltage Measurement/LConn2 -- -/RConn1
  Voltage Measurement/LConn1 -- +/RConn1

== system peripheral_utilities/SVPWM Modulation Module ==
  Ualpha : Inport
  Ubeta : Inport  Port=2
  Constant14 : Constant
  Constant15 : Constant
  Data Type Conversion : DataTypeConversion  OutDataTypeStr=uint32  SaturateOnIntegerOverflow=off  RndMeth=Floor
  Gain : Gain  Gain=half_cmp
  Mux3 : Mux  Inputs=3
  Saturation : Saturate  UpperLimit=1  LowerLimit=-1
  Subsystem : Subsystem
  Subsystem1 : Subsystem
  Subsystem2 : Subsystem
  sector : Subsystem
  Tabc : Outport
  wires:
  Subsystem/1(X) -> Subsystem1/2(X)
  Constant14/1 -> Subsystem2/4(Ts), Subsystem/4(Ts)
  Subsystem2/1(Ta) -> Mux3/1
  Subsystem2/3(Tc) -> Mux3/3
  Subsystem2/2(Tb) -> Mux3/2
  Ubeta/1 -> Subsystem/2(Ubeta), sector/2(Ubeta)
  sector/1(N) -> Subsystem2/1(N), Subsystem1/1(N)
  Subsystem1/1(T1) -> Subsystem2/2(T1)
  Ualpha/1 -> Subsystem/1(Ualpha), sector/1(Ualpha)
  Subsystem/2(Y) -> Subsystem1/3(Y)
  Subsystem1/2(T2) -> Subsystem2/3(T2)
  Subsystem/3(Z) -> Subsystem1/4(Z)
  Constant15/1 -> Subsystem/3(Udc)
  Mux3/1 -> Saturation/1
  Data Type Conversion/1 -> Tabc/1
  Gain/1 -> Data Type Conversion/1
  Saturation/1 -> Gain/1

== system peripheral_utilities/SVPWM Module(Ualpha-beta to Tabc, pu) ==
  Ualpha : Inport
  Ubeta : Inport  Port=2
  Constant : Constant  Value=half_cycle
  SVPWM Modulation : MATLAB Function  TreatAsAtomicUnit=on
  T : Outport
  wires:
  Constant/1 -> SVPWM Modulation/3(Half_cycle)
  Ualpha/1 -> SVPWM Modulation/1(Ualpha)
  Ubeta/1 -> SVPWM Modulation/2(Ubeta)
  SVPWM Modulation/1(T) -> T/1

== system peripheral_utilities/Single Phase Full Bridge ==
  Enable : Inport
  PWM CMP : Inport  Port=2
  MOSFET LOWER : spsMosfetLib/Mosfet  Ron=R_mosfet_on  Lon=Lon  Rd=Rd  Vfd=Vf  IC=0  Rs=Rs  Cs=Cs  Measurements=off
  MOSFET UPPER : spsMosfetLib/Mosfet  Ron=R_mosfet_on  Lon=Lon  Rd=Rd  Vfd=Vf  IC=0  Rs=Rs  Cs=Cs  Measurements=off
  Triangle PWM modulation (with deadband)1 : $bdroot/Triangle PWM modulation (with deadband)  fswitch=fswitch  CMP_MAX=CMP_MAX  Deadband_Upper=Deadband_Upper  Deadband_Lower=Deadband_Lower  phase_shift=phase_shift
  D : PMIOPort  Side=Left
  Phase : PMIOPort  Port=2  Side=Right
  S : PMIOPort  Port=3  Side=Right
  Sample Trigger Output : Outport
  wires:
  Triangle PWM modulation (with deadband)1/1 -> MOSFET UPPER/1
  Enable/1 -> Triangle PWM modulation (with deadband)1/1
  Triangle PWM modulation (with deadband)1/3 -> Sample Trigger Output/1
  Triangle PWM modulation (with deadband)1/2 -> MOSFET LOWER/1
  PWM CMP/1 -> Triangle PWM modulation (with deadband)1/2
  connections:
  MOSFET UPPER/LConn1 -- D/RConn1
  MOSFET LOWER/LConn1 -- Phase/RConn1 -- MOSFET UPPER/RConn1
  MOSFET LOWER/RConn1 -- S/RConn1

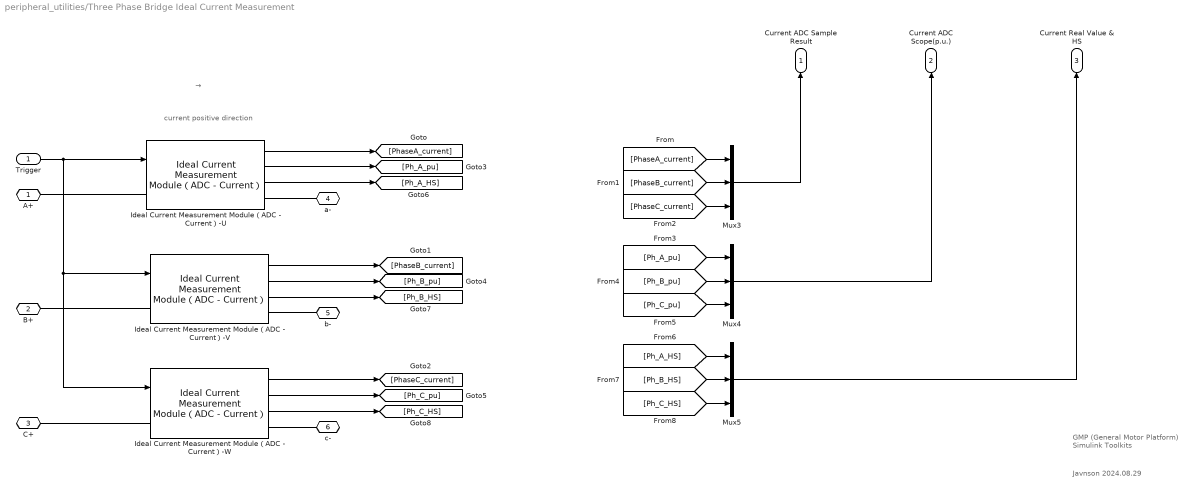
== system peripheral_utilities/Three Phase Bridge Ideal Current Measurement ==
  note: →
  note: Javnson
      | 2024.08.29
  note: GMP (General Motor Platform)
      | Simulink Toolkits
  note: current positive direction
  Trigger : Inport
  Ideal Current Measurement Module（ADC - Current）-U : $bdroot/Ideal Current Measurement Module（ADC - Current）  ADC_GAIN=ADC_GAIN  ADC_BIT=ADC_BIT  ADC_REFERENCE=ADC_REFERENCE  ADC_BIAS=ADC_BIAS  ADC_INIT=ADC_INIT
  Ideal Current Measurement Module（ADC - Current）-V : $bdroot/Ideal Current Measurement Module（ADC - Current）  ADC_GAIN=ADC_GAIN  ADC_BIT=ADC_BIT  ADC_REFERENCE=ADC_REFERENCE  ADC_BIAS=ADC_BIAS  ADC_INIT=ADC_INIT
  Ideal Current Measurement Module（ADC - Current）-W : $bdroot/Ideal Current Measurement Module（ADC - Current）  ADC_GAIN=ADC_GAIN  ADC_BIT=ADC_BIT  ADC_REFERENCE=ADC_REFERENCE  ADC_BIAS=ADC_BIAS  ADC_INIT=ADC_INIT
  Mux3 : Mux  Inputs=3
  Mux4 : Mux  Inputs=3
  Mux5 : Mux  Inputs=3
  A+ : PMIOPort  Side=Left
  B+ : PMIOPort  Port=2  Side=Left
  C+ : PMIOPort  Port=3  Side=Left
  a- : PMIOPort  Port=4  Side=Right
  b- : PMIOPort  Port=5  Side=Right
  c- : PMIOPort  Port=6  Side=Right
  Current ADC Sample Result : Outport
  Current ADC Scope(p.u.) : Outport  Port=2
  Current Real Value & HS : Outport  Port=3
  wires:
  [PhaseA_current] -> Mux3/1
  [PhaseB_current] -> Mux3/2
  [PhaseC_current] -> Mux3/3
  Mux3/1 -> Current ADC Sample Result/1
  [Ph_A_pu] -> Mux4/1
  [Ph_B_pu] -> Mux4/2
  [Ph_C_pu] -> Mux4/3
  Mux4/1 -> Current ADC Scope(p.u.)/1
  [Ph_B_HS] -> Mux5/2
  Mux5/1 -> Current Real Value & HS/1
  [Ph_C_HS] -> Mux5/3
  [Ph_A_HS] -> Mux5/1
  Trigger/1 -> Ideal Current Measurement Module（ADC - Current）-W/1, Ideal Current Measurement Module（ADC - Current）-V/1, Ideal Current Measurement Module（ADC - Current）-U/1
  Ideal Current Measurement Module（ADC - Current）-U/1 -> [PhaseA_current]
  Ideal Current Measurement Module（ADC - Current）-U/2 -> [Ph_A_pu]
  Ideal Current Measurement Module（ADC - Current）-U/3 -> [Ph_A_HS]
  Ideal Current Measurement Module（ADC - Current）-V/1 -> [PhaseB_current]
  Ideal Current Measurement Module（ADC - Current）-V/2 -> [Ph_B_pu]
  Ideal Current Measurement Module（ADC - Current）-V/3 -> [Ph_B_HS]
  Ideal Current Measurement Module（ADC - Current）-W/1 -> [PhaseC_current]
  Ideal Current Measurement Module（ADC - Current）-W/2 -> [Ph_C_pu]
  Ideal Current Measurement Module（ADC - Current）-W/3 -> [Ph_C_HS]
  connections:
  Ideal Current Measurement Module（ADC - Current）-U/LConn1 -- A+/RConn1
  Ideal Current Measurement Module（ADC - Current）-U/RConn1 -- a-/RConn1
  Ideal Current Measurement Module（ADC - Current）-V/RConn1 -- b-/RConn1
  Ideal Current Measurement Module（ADC - Current）-V/LConn1 -- B+/RConn1
  Ideal Current Measurement Module（ADC - Current）-W/RConn1 -- c-/RConn1
  Ideal Current Measurement Module（ADC - Current）-W/LConn1 -- C+/RConn1

== system peripheral_utilities/Three Phase Driver Model ==
  note: Javnson
      | 2024.08.29
  note: GMP (General Motor Platform)
      | Simulink Toolkits
  Enable : Inport
  PWM U : Inport  Port=2
  PWM V : Inport  Port=3
  PWM W : Inport  Port=4
  Single Phase Full Bridge U : $bdroot/Single Phase Full Bridge  fswitch=fswitch  CMP_MAX=CMP_MAX  Deadband_Upper=Deadband_Upper  Deadband_Lower=Deadband_Lower  Deadband_us=1  phase_shift=0  R_mosfet_on=R_mosfet_on  Lon=Lon  Rd=Rd  Vf=Vf  Rs=Rs  Cs=Cs
  Single Phase Full Bridge V : $bdroot/Single Phase Full Bridge  fswitch=fswitch  CMP_MAX=CMP_MAX  Deadband_Upper=Deadband_Upper  Deadband_Lower=Deadband_Lower  Deadband_us=1  phase_shift=0  R_mosfet_on=R_mosfet_on  Lon=Lon  Rd=Rd  Vf=Vf  Rs=Rs  Cs=Cs
  Single Phase Full Bridge W : $bdroot/Single Phase Full Bridge  fswitch=fswitch  CMP_MAX=CMP_MAX  Deadband_Upper=Deadband_Upper  Deadband_Lower=Deadband_Lower  Deadband_us=1  phase_shift=0  R_mosfet_on=R_mosfet_on  Lon=Lon  Rd=Rd  Vf=Vf  Rs=Rs  Cs=Cs
  Terminator : Terminator
  Terminator1 : Terminator
  U : PMIOPort  Side=Right
  V : PMIOPort  Port=2  Side=Right
  W : PMIOPort  Port=3  Side=Right
  Pwr+ : PMIOPort  Port=4  Side=Right
  Pwr- : PMIOPort  Port=5  Side=Right
  Sample Trigger Output : Outport
  wires:
  PWM W/1 -> Single Phase Full Bridge W/2
  Single Phase Full Bridge W/1 -> Terminator1/1
  Enable/1 -> Single Phase Full Bridge U/1, Single Phase Full Bridge W/1, Single Phase Full Bridge V/1
  Single Phase Full Bridge V/1 -> Terminator/1
  Single Phase Full Bridge U/1 -> Sample Trigger Output/1
  PWM U/1 -> Single Phase Full Bridge U/2
  PWM V/1 -> Single Phase Full Bridge V/2
  connections:
  Single Phase Full Bridge V/LConn1 -- Single Phase Full Bridge U/LConn1 -- Pwr+/RConn1 -- Single Phase Full Bridge W/LConn1
  Single Phase Full Bridge V/RConn2 -- Single Phase Full Bridge U/RConn2 -- Pwr-/RConn1 -- Single Phase Full Bridge W/RConn2
  Single Phase Full Bridge V/RConn1 -- V/RConn1
  Single Phase Full Bridge W/RConn1 -- W/RConn1
  Single Phase Full Bridge U/RConn1 -- U/RConn1
